simulink model "gm_Tx_OFDM"  (R2023a)
settings: Solver=FixedStepAuto  StartTime=0.0  StopTime=inf  RelTol=1e-3  EnableMultiTasking=on
model workspace (MAT data in the model file):
  M_ary = 16
  N = 64
  N_out = 256
  bit_per_symbol = 4
  fsc = 10000
  fsp = 640000
  stime = 0.0001
libraries: simulink x7, hdlmdlgenlib x4, dspsigops x4, hdlsllib x2, whdlmod x2, commdigbbndam3 x2, commrandsrc3 x1
settings Model: Creator=acer  LastModifiedBy=acer
settings SolverCC: AutoInsertRateTranBlk=on
settings OptimizationCC: BlockReduction=off  ConditionallyExecuteInputs=off  EnhancedBackFolding=on  PassReuseOutputArgsAs=Individual arguments  ZeroExternalMemoryAtStartup=off  ZeroInternalMemoryAtStartup=off  MaxStackSize=64  OptimizeBlockOrder=speed  DifferentSizesBufferReuse=on  OptimizationCustomize=off  EfficientTunableParamExpr=on
settings DebuggingCC: InheritedTsInSrcMsg=none  SingleTaskRateTransMsg=error  ParameterTunabilityLossMsg=error
settings HardwareCC: ProdBitPerPointer=32  ProdBitPerSizeT=32  ProdBitPerPtrDiffT=32  ProdLargestAtomicInteger=Long  ProdLargestAtomicFloat=Double  ProdWordSize=32  ProdHWDeviceType=ARM Compatible->ARM Cortex
settings SFSimCC: MATLABDynamicMemAlloc=off
settings RTWCC: Description=Embedded Coder  SystemTargetFile=ert.tlc  TLCOptions="-aInlineSetEventsForThisBaseRateFcn=TLC_FALSE -aSuppressMultiTaskScheduler=TLC_FALSE  -aRateBasedStepFcn=0"  TemplateMakefile=ert_default_tmf
settings CodeAppCC: ForceParamTrailComments=on  IgnoreCustomStorageClasses=off  OperatorAnnotations=on  SimulinkDataObjDesc=on  SFDataObjDesc=on  InsertBlockDesc=on

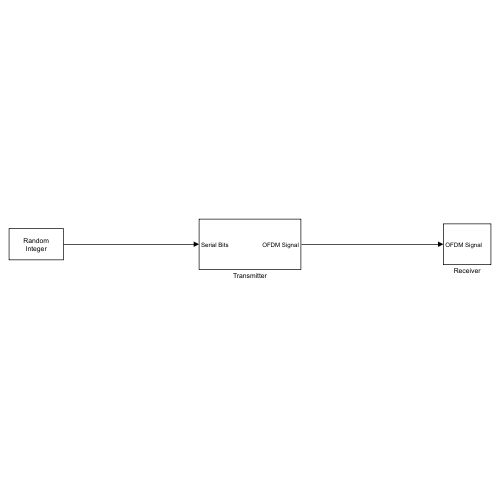
[thumbnail: Simulink's stored preview of the top-level diagram]
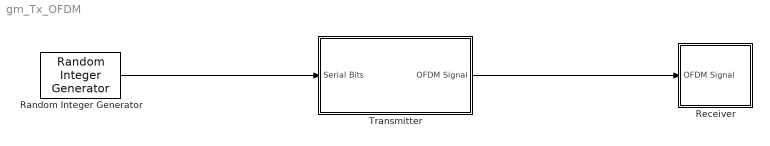
== system gm_Tx_OFDM ==
  Random Integer Generator : commrandsrc3/Random Integer Generator  SetSize=16  SeedSource=Auto  Seed=0  SampleTime=stime  SamplesPerFrame=1  OutputDataType=uint8  SimulateUsing=Interpreted execution
  Receiver : Subsystem
  Transmitter : Subsystem
  wires:
  Random Integer Generator/1 -> Transmitter/1(Serial Bits)
  Transmitter/1(OFDM Signal) -> Receiver/1(OFDM Signal)

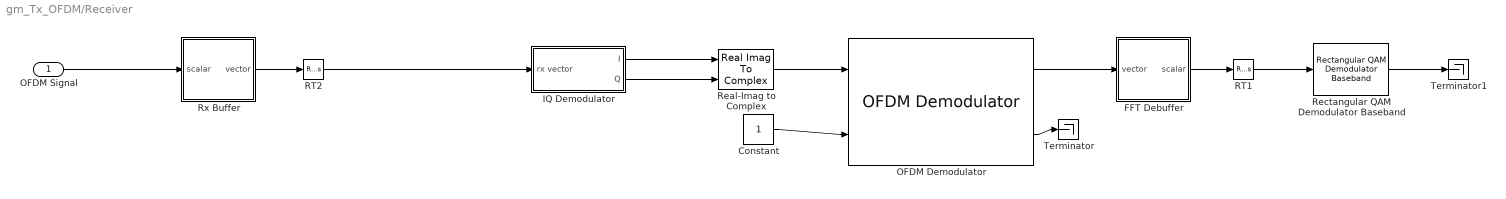
== system gm_Tx_OFDM/Receiver ==
  OFDM Signal : Inport
  Constant : Constant  OutDataTypeStr=boolean  SampleTime=-1
  FFT Debuffer : Subsystem
  IQ Demodulator : Subsystem
  OFDM Demodulator : whdlmod/OFDM Demodulator  OFDMParamsSource=Property  MaxFFTLength=64  FFTLength=N*2  CPLength=32  NumLGsC=16  NumRGsC=15  CPFraction=off  CPFractionSource=Property  CPFractionValue=0.55  removeDCSubcarriers=on  enableResetInputPort=off  Normalize=off  RoundingMethod=Floor  SimulateUsing=Code generation
  RT1 : RateTransition  OutPortSampleTime=stime/N
  RT2 : RateTransition  OutPortSampleTime=stime
  Real-Imag to Complex : RealImagToComplex
  Rectangular QAM Demodulator Baseband : commdigbbndam3/Rectangular QAM Demodulator Baseband  M=16  OutType=Integer  DecType=Hard decision  VarSource=Dialog  Variance=1  Dec=Gray  Mapping=[0:15]  PowType=Min. distance between symbols  MinDist=2  AvgPow=1  PeakPow=1  Ph=0  outDtype1=Inherit via internal rule  outDtype2=Inherit via internal rule  derotateFactorWordLen=16  derotateFactorDataTypeStr=Inherit: Same word length as input  derotateFactorLastDataTypeStr=Inherit: Same word length as input  denormFactorWordLen=16  denormFactorDataTypeStr=Inherit: Same word length as input  denormFactorLastDataTypeStr=Inherit: Same word length as input  prodOutWordLen=32  prodOutOverflowMode=Wrap  prodOutRoundingMode=Floor  prodOutOvFlMode=off  prodOutOvFlModeLastStrValue=off  sumWordLen=32
      settings: LibrarySourceBlock=|
      | commhdldigbbndam/Rectangular QAM
      | Demodulator
      | Baseband
  Rx Buffer : Subsystem
  Terminator : Terminator
  Terminator1 : Terminator
  wires:
  IQ Demodulator/2(Q) -> Real-Imag to Complex/2
  IQ Demodulator/1(I) -> Real-Imag to Complex/1
  RT2/1 -> IQ Demodulator/1(rx vector)
  Rectangular QAM Demodulator Baseband/1 -> Terminator1/1
  RT1/1 -> Rectangular QAM Demodulator Baseband/1
  FFT Debuffer/1(scalar) -> RT1/1
  OFDM Demodulator/1 -> FFT Debuffer/1(vector)
  OFDM Demodulator/2 -> Terminator/1
  Constant/1 -> OFDM Demodulator/2
  Real-Imag to Complex/1 -> OFDM Demodulator/1
  Rx Buffer/1(vector) -> RT2/1
  OFDM Signal/1 -> Rx Buffer/1(scalar)

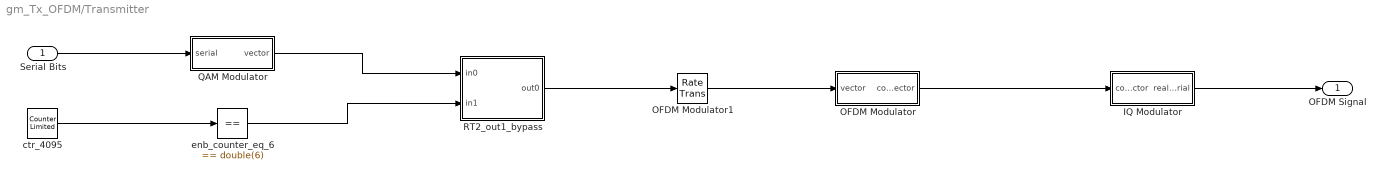
== system gm_Tx_OFDM/Transmitter ==
  Serial Bits : Inport  OutDataTypeStr=uint8  PortDimensions=1  SampleTime=0.0001
  IQ Modulator : Subsystem
  OFDM Modulator : Subsystem
  OFDM Modulator1 : RateTransition  OutPortSampleTimeOpt=Multiple of input port sample time  OutPortSampleTimeMultiple=4096
  QAM Modulator : Subsystem
  RT2_out1_bypass : Subsystem
  ctr_4095 : simulink/Sources/Counter Limited  uplimit=double(4095)  tsamp=1.5625e-06
  enb_counter_eq_6 : simulink/Logic and Bit Operations/Compare To Constant  relop===  const=double(6)  OutDataTypeStr=boolean
  OFDM Signal : Outport  SampleTime=1.5625e-06
  wires:
  Serial Bits/1 -> QAM Modulator/1(serial)
  IQ Modulator/1(real_serial) -> OFDM Signal/1
  OFDM Modulator/1(complex_vector) -> IQ Modulator/1(complex_vector)
  QAM Modulator/1(vector) -> RT2_out1_bypass/1(in0)
  OFDM Modulator1/1 -> OFDM Modulator/1(vector)
  RT2_out1_bypass/1(out0) -> OFDM Modulator1/1
  enb_counter_eq_6/1 -> RT2_out1_bypass/2(in1)
  ctr_4095/1 -> enb_counter_eq_6/1

== system gm_Tx_OFDM/Receiver/FFT Debuffer ==
  note: When changing N, change the vector init size to N manually
  vector : Inport
  Data Type Conversion : DataTypeConversion  OutMin=0  OutMax=1  OutDataTypeStr=fixdt(1,16)  SaturateOnIntegerOverflow=off  RndMeth=Floor
  Data Type Conversion1 : DataTypeConversion  OutMin=0  OutMax=1  OutDataTypeStr=fixdt(1,16)  SaturateOnIntegerOverflow=off  RndMeth=Floor
  Delay : Delay  DelayLength=1
  HDL Counter : hdlsllib/Sources/HDL Counter  CountType=Count limited  CountInit=1  CountStep=1  CountMax=N  CountFromType=Initial value  CountFrom=1  CountResetPort=off  CountLoadPort=off  CountEnbPort=off  CountDirPort=off  CountHitOutputPort=off  CountDataType=Signed  CountWordLen=16  CountFracLen=0  CountSampTime=stime
  debuffer : MATLAB Function  TreatAsAtomicUnit=on
  vector feedback : MATLAB Function  TreatAsAtomicUnit=on
  scalar : Outport
  wires:
  Data Type Conversion1/1 -> debuffer/1(vector_in)
  vector/1 -> Data Type Conversion1/1
  Delay/1 -> vector feedback/1(vector_before)
  vector feedback/1(y) -> Data Type Conversion/1
  debuffer/2(vector_current) -> Delay/1
  Data Type Conversion/1 -> debuffer/3(vector_before)
  HDL Counter/1 -> debuffer/2(counter)
  debuffer/1(buffer) -> scalar/1

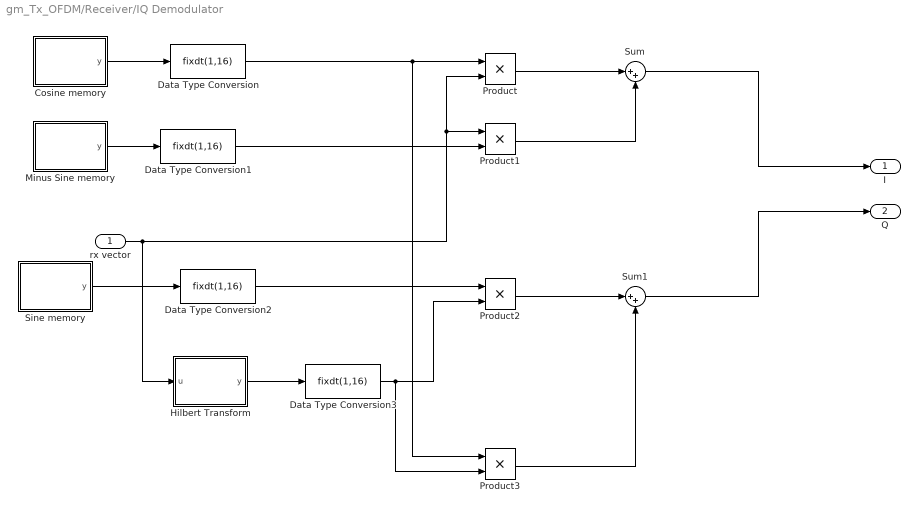
== system gm_Tx_OFDM/Receiver/IQ Demodulator ==
  rx vector : Inport
  Cosine memory : MATLAB Function  TreatAsAtomicUnit=on
  Data Type Conversion{,1..3} (4 alike) : DataTypeConversion  OutMin=0  OutMax=1  OutDataTypeStr=fixdt(1,16)  SaturateOnIntegerOverflow=off  RndMeth=Floor
  Hilbert Transform : MATLAB Function  TreatAsAtomicUnit=on
  Minus Sine memory : MATLAB Function  TreatAsAtomicUnit=on
  Product{,1..3} (4 alike) : Product
  Sine memory : MATLAB Function  TreatAsAtomicUnit=on
  Sum : Sum  Inputs=|++
  Sum1 : Sum  Inputs=|++
  I : Outport
  Q : Outport  Port=2
  wires:
  Data Type Conversion3/1 -> Product2/2, Product3/2
  Hilbert Transform/1(y) -> Data Type Conversion3/1
  Data Type Conversion2/1 -> Product2/1
  Sine memory/1(y) -> Data Type Conversion2/1
  Data Type Conversion1/1 -> Product1/2
  Minus Sine memory/1(y) -> Data Type Conversion1/1
  Data Type Conversion/1 -> Product/1, Product3/1
  Cosine memory/1(y) -> Data Type Conversion/1
  Sum/1 -> I/1
  Product3/1 -> Sum1/2
  Product2/1 -> Sum1/1
  Product/1 -> Sum/1
  Product1/1 -> Sum/2
  rx vector/1 -> Hilbert Transform/1(u), Product/2, Product1/1
  Sum1/1 -> Q/1

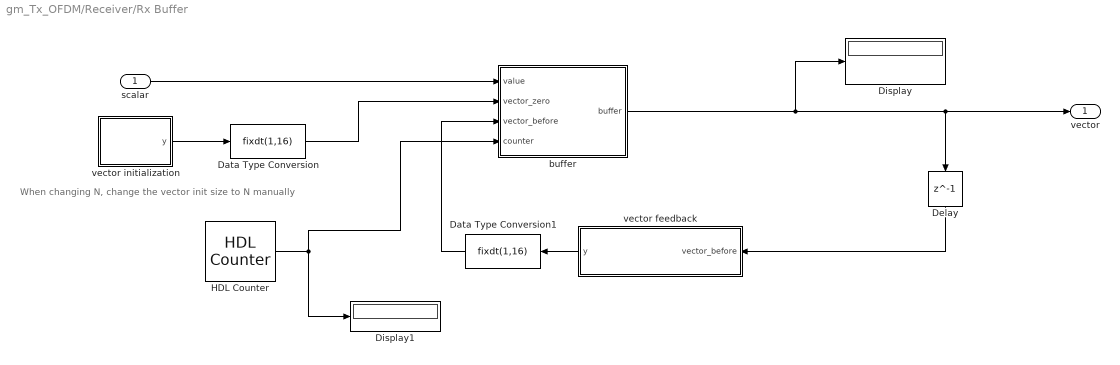
== system gm_Tx_OFDM/Receiver/Rx Buffer ==
  note: When changing N, change the vector init size to N manually
  scalar : Inport
  Data Type Conversion : DataTypeConversion  OutMin=0  OutMax=1  OutDataTypeStr=fixdt(1,16)  SaturateOnIntegerOverflow=off  RndMeth=Floor
  Data Type Conversion1 : DataTypeConversion  OutMin=0  OutMax=1  OutDataTypeStr=fixdt(1,16)  SaturateOnIntegerOverflow=off  RndMeth=Floor
  Delay : Delay  DelayLength=1
  Display : Display
  Display1 : Display
  HDL Counter : hdlsllib/Sources/HDL Counter  CountType=Count limited  CountInit=1  CountStep=1  CountMax=N  CountFromType=Initial value  CountFrom=1  CountResetPort=off  CountLoadPort=off  CountEnbPort=off  CountDirPort=off  CountHitOutputPort=off  CountDataType=Unsigned  CountWordLen=16  CountFracLen=0  CountSampTime=stime/N
  buffer : MATLAB Function  TreatAsAtomicUnit=on
  vector feedback : MATLAB Function  TreatAsAtomicUnit=on
  vector initialization : MATLAB Function  TreatAsAtomicUnit=on
  vector : Outport
  wires:
  HDL Counter/1 -> Display1/1, buffer/4(counter)
  scalar/1 -> buffer/1(value)
  Data Type Conversion1/1 -> buffer/3(vector_before)
  vector feedback/1(y) -> Data Type Conversion1/1
  Delay/1 -> vector feedback/1(vector_before)
  buffer/1(buffer) -> vector/1, Delay/1, Display/1
  Data Type Conversion/1 -> buffer/2(vector_zero)
  vector initialization/1(y) -> Data Type Conversion/1

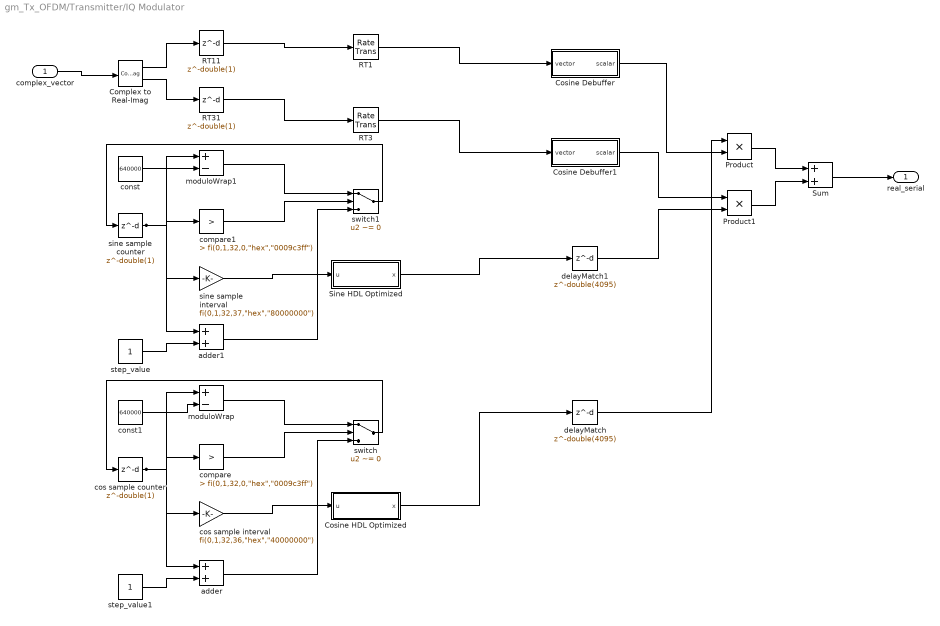
== system gm_Tx_OFDM/Transmitter/IQ Modulator ==
  complex_vector : Inport  OutDataTypeStr=fixdt(1, 16, 14)  PortDimensions=[64 1]  SampleTime=0.0064
      settings: SignalType=complex
  Complex to Real-Imag : ComplexToRealImag  SampleTime=0.0064
  Cosine Debuffer : Subsystem
  Cosine Debuffer1 : Subsystem
  Cosine HDL Optimized : Subsystem  mask(Sine and Cosine HDL optimized block){OutputFormula=cos(2*pi*u), NumDataPoints=double(64), TableDataTypeStr=fixdt(0,16,15), SimulateLUTROMDelay=off}
      mask prompts: OutputFormula "Simulink:masks:OutputFormula_MP"; NumDataPoints "HDLShared:hdlshared:CosineHDL_Npts"; TableDataTypeStr "Simulink:blkprm_prompts:TABLE_UNIFIEDDATATYPE"; SimulateLUTROMDelay "HDLShared:hdlshared:CosineHDL_SimulateLUTDelay"
      mask help: Sine and Cosine HDL optimized block using quarter wave symmetry, and HDL friendly settings.
      mask Help: helpview([docroot '/hdlcoder/helptargets.map'],'SineAndCosineHDL_Optimized');
      mask TypeOptions OutputFormula: sin(2*pi*u) | cos(2*pi*u) | exp(j*2*pi*u) | sin(2*pi*u) and cos(2*pi*u)
      mask Display:
      | port_label('input',1,'u')
      | port_label('output',1,'cos(2*pi*u)')
      | xpos = 0.35;
      | yoffset = 0.5;
      | if ( SimulateLUTROMDelay )
      |   text(xpos,yoffset,'HDL (Z^{-1})','texmode','on')
      | else
      |    text(xpos,yoffset,'HDL')
      | end
  Product : Product  Inputs=**  OutDataTypeStr=fixdt(1, 33, 29)  SampleTime=1.5625e-06
  Product1 : Product  Inputs=**  OutDataTypeStr=int16  SampleTime=1.5625e-06
  RT1 : RateTransition  Integrity=off  Deterministic=off  InitialCondition=double(0)  OutPortSampleTimeOpt=Multiple of input port sample time  OutPortSampleTimeMultiple=1/4096
  RT11 : Delay  DelayLength=double(1)  InitialCondition=0  SampleTime=0.0064
  RT3 : RateTransition  Integrity=off  Deterministic=off  InitialCondition=double(0)  OutPortSampleTimeOpt=Multiple of input port sample time  OutPortSampleTimeMultiple=1/4096
  RT31 : Delay  DelayLength=double(1)  InitialCondition=0  SampleTime=0.0064
  Sine HDL Optimized : Subsystem  mask(Sine and Cosine HDL optimized block){OutputFormula=sin(2*pi*u), NumDataPoints=double(64), TableDataTypeStr=fixdt(0,16,15), SimulateLUTROMDelay=off}
      mask prompts: OutputFormula "Simulink:masks:OutputFormula_MP"; NumDataPoints "HDLShared:hdlshared:CosineHDL_Npts"; TableDataTypeStr "Simulink:blkprm_prompts:TABLE_UNIFIEDDATATYPE"; SimulateLUTROMDelay "HDLShared:hdlshared:CosineHDL_SimulateLUTDelay"
      mask help: Sine and Cosine HDL optimized block using quarter wave symmetry, and HDL friendly settings.
      mask Help: helpview([docroot '/hdlcoder/helptargets.map'],'SineAndCosineHDL_Optimized');
      mask TypeOptions OutputFormula: sin(2*pi*u) | cos(2*pi*u) | exp(j*2*pi*u) | sin(2*pi*u) and cos(2*pi*u)
      mask Display:
      | port_label('input',1,'u')
      | port_label('output',1,'sin(2*pi*u)')
      | xpos = 0.35;
      | yoffset = 0.5;
      | if ( SimulateLUTROMDelay )
      |   text(xpos,yoffset,'HDL (Z^{-1})','texmode','on')
      | else
      |    text(xpos,yoffset,'HDL')
      | end
  Sum : Sum  AccumDataTypeStr=fixdt(1, 64, 29)  OutDataTypeStr=fixdt(1, 64, 29)  SampleTime=1.5625e-06
  adder : Sum  AccumDataTypeStr=int32  OutDataTypeStr=int32  SampleTime=1.5625e-06
  adder1 : Sum  AccumDataTypeStr=int32  OutDataTypeStr=int32  SampleTime=1.5625e-06
  compare : simulink/Logic and Bit Operations/Compare To Constant  relop=>  const="fi(0,1,32,0,\"hex\",\"0009c3ff\")"  OutDataTypeStr=boolean
  compare1 : simulink/Logic and Bit Operations/Compare To Constant  relop=>  const="fi(0,1,32,0,\"hex\",\"0009c3ff\")"  OutDataTypeStr=boolean
  const : Constant  Value=640000  VectorParams1D=off  OutDataTypeStr=int32  SampleTime=1.5625e-06
  const1 : Constant  Value=640000  VectorParams1D=off  OutDataTypeStr=int32  SampleTime=1.5625e-06
  cos sample counter : Delay  DelayLength=double(1)  InitialCondition=0  SampleTime=1.5625e-06
  cos sample interval : Gain  Gain="fi(0,1,32,36,\"hex\",\"40000000\")"  ParamDataTypeStr=fixdt(1, 32, 36)  OutDataTypeStr=fixdt(1, 64, 36)  SampleTime=1.5625e-06
  delayMatch : Delay  DelayLength=double(4095)  InitialCondition=0  SampleTime=1.5625e-06
  delayMatch1 : Delay  DelayLength=double(4095)  InitialCondition=0  SampleTime=1.5625e-06
  moduloWrap : Sum  Inputs=+-  AccumDataTypeStr=int32  OutDataTypeStr=int32  SampleTime=1.5625e-06
  moduloWrap1 : Sum  Inputs=+-  AccumDataTypeStr=int32  OutDataTypeStr=int32  SampleTime=1.5625e-06
  sine sample counter : Delay  DelayLength=double(1)  InitialCondition=0  SampleTime=1.5625e-06
  sine sample interval : Gain  Gain="fi(0,1,32,37,\"hex\",\"80000000\")"  ParamDataTypeStr=fixdt(1, 32, 37)  OutDataTypeStr=fixdt(1, 64, 37)  SampleTime=1.5625e-06
  step_value : Constant  VectorParams1D=off  OutDataTypeStr=int32  SampleTime=1.5625e-06
  step_value1 : Constant  VectorParams1D=off  OutDataTypeStr=int32  SampleTime=1.5625e-06
  switch : Switch  Criteria=u2 ~= 0  Threshold=double(0)  OutDataTypeStr=int32  SampleTime=1.5625e-06  SaturateOnIntegerOverflow=off  InputSameDT=off
  switch1 : Switch  Criteria=u2 ~= 0  Threshold=double(0)  OutDataTypeStr=int32  SampleTime=1.5625e-06  SaturateOnIntegerOverflow=off  InputSameDT=off
  real_serial : Outport  SampleTime=1.5625e-06
  wires:
  Cosine Debuffer/1(scalar) -> Product/2
  Cosine Debuffer1/1(scalar) -> Product1/1
  Sum/1 -> real_serial/1
  cos sample counter/1 -> cos sample interval/1, compare/1, moduloWrap/1, adder/1
  sine sample counter/1 -> sine sample interval/1, compare1/1, moduloWrap1/1, adder1/1
  RT1/1 -> Cosine Debuffer/1(vector)
  RT3/1 -> Cosine Debuffer1/1(vector)
  RT11/1 -> RT1/1
  RT31/1 -> RT3/1
  sine sample interval/1 -> Sine HDL Optimized/1(u)
  delayMatch1/1 -> Product1/2
  Product1/1 -> Sum/2
  Product/1 -> Sum/1
  cos sample interval/1 -> Cosine HDL Optimized/1(u)
  delayMatch/1 -> Product/1
  const/1 -> moduloWrap1/2
  step_value/1 -> adder1/2
  const1/1 -> moduloWrap/2
  step_value1/1 -> adder/2
  Complex to Real-Imag/1 -> RT11/1
  Complex to Real-Imag/2 -> RT31/1
  complex_vector/1 -> Complex to Real-Imag/1
  Cosine HDL Optimized/1(x) -> delayMatch/1
  Sine HDL Optimized/1(x) -> delayMatch1/1
  switch1/1 -> sine sample counter/1
  adder1/1 -> switch1/3
  compare1/1 -> switch1/2
  moduloWrap1/1 -> switch1/1
  switch/1 -> cos sample counter/1
  adder/1 -> switch/3
  compare/1 -> switch/2
  moduloWrap/1 -> switch/1

== system gm_Tx_OFDM/Transmitter/OFDM Modulator ==
  vector : Inport  OutDataTypeStr=fixdt(1, 16, 14)  PortDimensions=[64]  SampleTime=0.0064
      settings: SignalType=complex
  Constant : Constant  OutDataTypeStr=boolean  SampleTime=0.0064
  OFDM Modulator : Subsystem
  complex_vector : Outport  SampleTime=0.0064
  wires:
  Constant/1 -> OFDM Modulator/2(valid)
  OFDM Modulator/1(data1) -> complex_vector/1
  vector/1 -> OFDM Modulator/1(data)

== system gm_Tx_OFDM/Transmitter/QAM Modulator ==
  note: When changing N, change the vector init size to N manually
  serial : Inport  OutDataTypeStr=uint8  PortDimensions=1  SampleTime=0.0001
  QAM Buffer : Subsystem
  Rectangular QAM Modulator Baseband : commdigbbndam3/Rectangular QAM Modulator Baseband  M=M_ary  InType=Integer  Enc=Gray  Mapping=[0:15]  PowType=Min. distance between symbols  MinDist=2  AvgPow=1  PeakPow=1  Ph=0  outDtype=Fixed-point  outWordLen=16  outUDDataType=sfix(16)  outFracLenMode=Best precision  outFracLen=15  outDataTypeStr=fixdt(1,16)  outLastDataTypeStr=fixdt(1,16)
      settings: LibrarySourceBlock=|
      | commhdldigbbndam/Rectangular QAM
      | Modulator
      | Baseband
  vector : Outport  SampleTime=1.5625e-06
  wires:
  Rectangular QAM Modulator Baseband/1 -> QAM Buffer/1(scalar)
  QAM Buffer/1(vector) -> vector/1
  serial/1 -> Rectangular QAM Modulator Baseband/1

== system gm_Tx_OFDM/Transmitter/RT2_out1_bypass ==
  in0 : Inport  OutDataTypeStr=fixdt(1,16,14,'DataTypeOverride', 'Off')  PortDimensions=[64]  SampleTime=1.5625e-06
      settings: SignalType=complex
  in1 : Inport  Port=2  OutDataTypeStr=boolean  SampleTime=1.5625e-06
  RT2_out1_enb : Switch  Criteria=u2 ~= 0  Threshold=double(0)  OutDataTypeStr=fixdt(1, 16, 14)  SampleTime=1.5625e-06  SaturateOnIntegerOverflow=off  InputSameDT=off
  RT2_out1_state : Delay  DelayLength=double(1)  InitialCondition=0  SampleTime=1.5625e-06
  out0 : Outport  OutDataTypeStr=fixdt(1, 16, 14)  PortDimensions=[64]  SampleTime=1.5625e-06
      settings: SignalType=complex
  wires:
  RT2_out1_enb/1 -> out0/1, RT2_out1_state/1
  in0/1 -> RT2_out1_enb/1
  in1/1 -> RT2_out1_enb/2
  RT2_out1_state/1 -> RT2_out1_enb/3

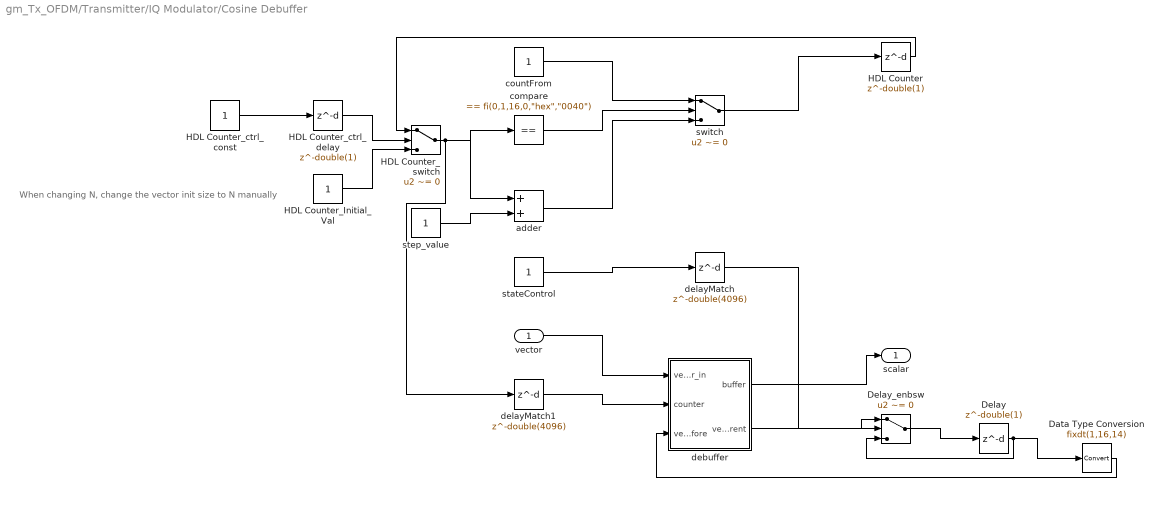
== system gm_Tx_OFDM/Transmitter/IQ Modulator/Cosine Debuffer ==
  note: When changing N, change the vector init size to N manually
  vector : Inport  OutDataTypeStr=fixdt(1, 16, 14)  PortDimensions=[64 1]  SampleTime=1.5625e-06
  Data Type Conversion : DataTypeConversion  OutDataTypeStr=fixdt(1,16,14)
  Delay : Delay  DelayLength=double(1)  InitialCondition=0  SampleTime=1.5625e-06
  Delay_enbsw : Switch  Criteria=u2 ~= 0  Threshold=double(0)  OutDataTypeStr=fixdt(1, 16, 14)  SampleTime=1.5625e-06  SaturateOnIntegerOverflow=off  InputSameDT=off
  HDL Counter : Delay  DelayLength=double(1)  InitialCondition=0  SampleTime=1.5625e-06
  HDL Counter_Initial_Val : Constant  OutDataTypeStr=int16  SampleTime=1.5625e-06
  HDL Counter_ctrl_const : Constant  OutDataTypeStr=boolean  SampleTime=1.5625e-06
  HDL Counter_ctrl_delay : Delay  DelayLength=double(1)  InitialCondition=0  SampleTime=1.5625e-06
  HDL Counter_switch : Switch  Criteria=u2 ~= 0  Threshold=double(0)  OutDataTypeStr=int16  SampleTime=1.5625e-06  SaturateOnIntegerOverflow=off  InputSameDT=off
  adder : Sum  AccumDataTypeStr=int16  OutDataTypeStr=int16  SampleTime=1.5625e-06
  compare : simulink/Logic and Bit Operations/Compare To Constant  relop===  const="fi(0,1,16,0,\"hex\",\"0040\")"  OutDataTypeStr=boolean
  countFrom : Constant  VectorParams1D=off  OutDataTypeStr=int16  SampleTime=1.5625e-06
  debuffer : Subsystem
  delayMatch : Delay  DelayLength=double(4096)  InitialCondition=0  SampleTime=1.5625e-06
  delayMatch1 : Delay  DelayLength=double(4096)  InitialCondition=0  SampleTime=1.5625e-06
  stateControl : Constant  OutDataTypeStr=boolean  SampleTime=1.5625e-06
  step_value : Constant  VectorParams1D=off  OutDataTypeStr=int16  SampleTime=1.5625e-06
  switch : Switch  Criteria=u2 ~= 0  Threshold=double(0)  OutDataTypeStr=int16  SampleTime=1.5625e-06  SaturateOnIntegerOverflow=off  InputSameDT=off
  scalar : Outport  SampleTime=1.5625e-06
  wires:
  delayMatch1/1 -> debuffer/2(counter)
  step_value/1 -> adder/2
  countFrom/1 -> switch/1
  HDL Counter_Initial_Val/1 -> HDL Counter_switch/3
  HDL Counter_ctrl_const/1 -> HDL Counter_ctrl_delay/1
  HDL Counter_ctrl_delay/1 -> HDL Counter_switch/2
  delayMatch/1 -> Delay_enbsw/2
  vector/1 -> debuffer/1(vector_in)
  stateControl/1 -> delayMatch/1
  HDL Counter_switch/1 -> delayMatch1/1, adder/1, compare/1
  HDL Counter/1 -> HDL Counter_switch/1
  switch/1 -> HDL Counter/1
  adder/1 -> switch/3
  compare/1 -> switch/2
  Delay/1 -> Data Type Conversion/1, Delay_enbsw/3
  Data Type Conversion/1 -> debuffer/3(vector_before)
  debuffer/2(vector_current) -> Delay_enbsw/1
  debuffer/1(buffer) -> scalar/1
  Delay_enbsw/1 -> Delay/1

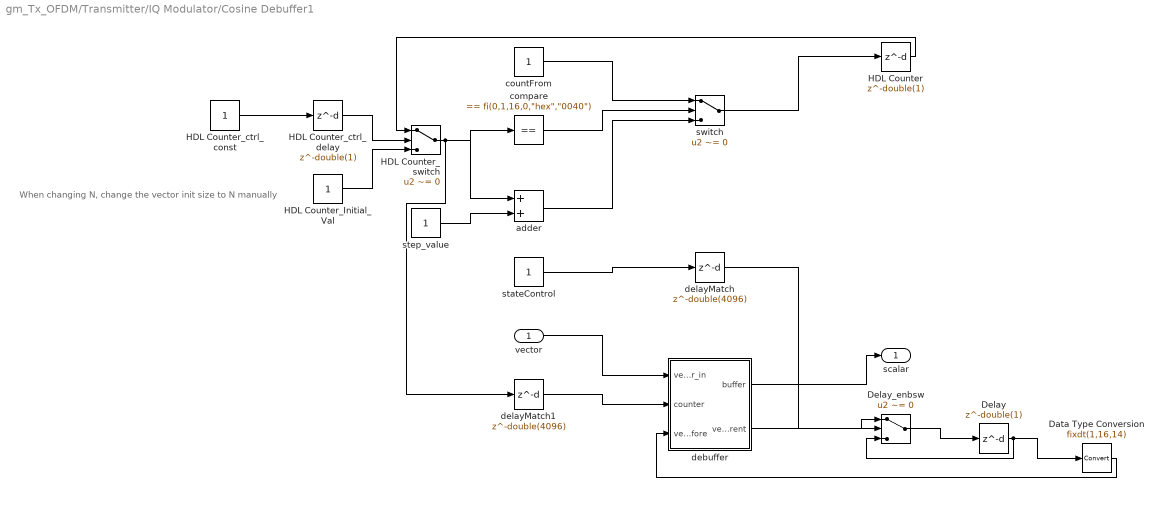
== system gm_Tx_OFDM/Transmitter/IQ Modulator/Cosine Debuffer1 ==
  note: When changing N, change the vector init size to N manually
  vector : Inport  OutDataTypeStr=fixdt(1, 16, 14)  PortDimensions=[64 1]  SampleTime=1.5625e-06
  Data Type Conversion : DataTypeConversion  OutDataTypeStr=fixdt(1,16,14)
  Delay : Delay  DelayLength=double(1)  InitialCondition=0  SampleTime=1.5625e-06
  Delay_enbsw : Switch  Criteria=u2 ~= 0  Threshold=double(0)  OutDataTypeStr=fixdt(1, 16, 14)  SampleTime=1.5625e-06  SaturateOnIntegerOverflow=off  InputSameDT=off
  HDL Counter : Delay  DelayLength=double(1)  InitialCondition=0  SampleTime=1.5625e-06
  HDL Counter_Initial_Val : Constant  OutDataTypeStr=int16  SampleTime=1.5625e-06
  HDL Counter_ctrl_const : Constant  OutDataTypeStr=boolean  SampleTime=1.5625e-06
  HDL Counter_ctrl_delay : Delay  DelayLength=double(1)  InitialCondition=0  SampleTime=1.5625e-06
  HDL Counter_switch : Switch  Criteria=u2 ~= 0  Threshold=double(0)  OutDataTypeStr=int16  SampleTime=1.5625e-06  SaturateOnIntegerOverflow=off  InputSameDT=off
  adder : Sum  AccumDataTypeStr=int16  OutDataTypeStr=int16  SampleTime=1.5625e-06
  compare : simulink/Logic and Bit Operations/Compare To Constant  relop===  const="fi(0,1,16,0,\"hex\",\"0040\")"  OutDataTypeStr=boolean
  countFrom : Constant  VectorParams1D=off  OutDataTypeStr=int16  SampleTime=1.5625e-06
  debuffer : Subsystem
  delayMatch : Delay  DelayLength=double(4096)  InitialCondition=0  SampleTime=1.5625e-06
  delayMatch1 : Delay  DelayLength=double(4096)  InitialCondition=0  SampleTime=1.5625e-06
  stateControl : Constant  OutDataTypeStr=boolean  SampleTime=1.5625e-06
  step_value : Constant  VectorParams1D=off  OutDataTypeStr=int16  SampleTime=1.5625e-06
  switch : Switch  Criteria=u2 ~= 0  Threshold=double(0)  OutDataTypeStr=int16  SampleTime=1.5625e-06  SaturateOnIntegerOverflow=off  InputSameDT=off
  scalar : Outport  SampleTime=1.5625e-06
  wires:
  delayMatch1/1 -> debuffer/2(counter)
  step_value/1 -> adder/2
  countFrom/1 -> switch/1
  HDL Counter_Initial_Val/1 -> HDL Counter_switch/3
  HDL Counter_ctrl_const/1 -> HDL Counter_ctrl_delay/1
  HDL Counter_ctrl_delay/1 -> HDL Counter_switch/2
  delayMatch/1 -> Delay_enbsw/2
  vector/1 -> debuffer/1(vector_in)
  stateControl/1 -> delayMatch/1
  HDL Counter_switch/1 -> delayMatch1/1, adder/1, compare/1
  HDL Counter/1 -> HDL Counter_switch/1
  switch/1 -> HDL Counter/1
  adder/1 -> switch/3
  compare/1 -> switch/2
  Delay/1 -> Data Type Conversion/1, Delay_enbsw/3
  Data Type Conversion/1 -> debuffer/3(vector_before)
  debuffer/2(vector_current) -> Delay_enbsw/1
  debuffer/1(buffer) -> scalar/1
  Delay_enbsw/1 -> Delay/1

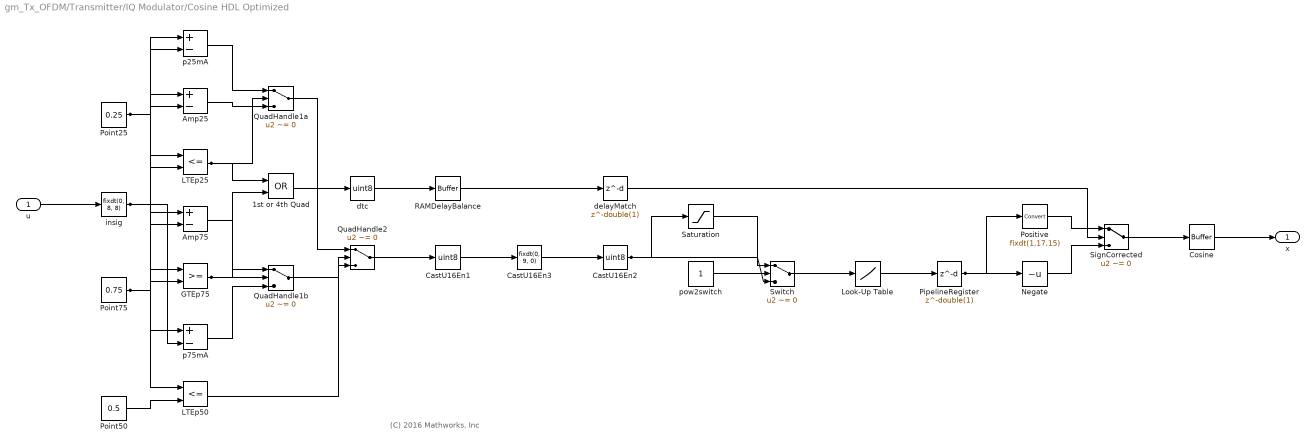
== system gm_Tx_OFDM/Transmitter/IQ Modulator/Cosine HDL Optimized ==
  note: (C) 2016 Mathworks, Inc
  u : Inport  OutDataTypeStr=fixdt(1,64,36,'DataTypeOverride', 'Off')  SampleTime=1.5625e-06
  1st or 4th Quad : Logic  Operator=OR  AllPortsSameDT=off  OutDataTypeStr=boolean  SampleTime=1.5625e-06
  Amp25 : Sum  Inputs=+-  AccumDataTypeStr=fixdt(1, 32, 17)  OutDataTypeStr=fixdt(0, 32, 17)  SampleTime=1.5625e-06
  Amp75 : Sum  Inputs=+-  AccumDataTypeStr=fixdt(1, 32, 17)  OutDataTypeStr=fixdt(0, 32, 17)  SampleTime=1.5625e-06
  CastU16En1 : DataTypeConversion  OutDataTypeStr=uint8  ConvertRealWorld=Stored Integer (SI)  SampleTime=1.5625e-06  SaturateOnIntegerOverflow=off  RndMeth=Floor
  CastU16En2 : DataTypeConversion  OutDataTypeStr=uint8  ConvertRealWorld=Stored Integer (SI)  SampleTime=1.5625e-06  RndMeth=Floor
  CastU16En3 : DataTypeConversion  OutDataTypeStr=fixdt(0, 9, 0)  SampleTime=1.5625e-06  SaturateOnIntegerOverflow=off  RndMeth=Floor
  Cosine : hdlmdlgenlib/Buffer
  GTEp75 : RelationalOperator  OutDataTypeStr=boolean  SampleTime=1.5625e-06  InputSameDT=off
  LTEp25 : RelationalOperator  Operator=<=  OutDataTypeStr=boolean  SampleTime=1.5625e-06  InputSameDT=off
  LTEp50 : RelationalOperator  Operator=<=  OutDataTypeStr=boolean  SampleTime=1.5625e-06  InputSameDT=off
  Look-Up Table : Lookup_n-D  NumberOfTableDimensions=1  BreakpointsForDimension1="fi(\"numerictype\",numerictype(0,8,0),\"fimath\",fimath(\"RoundingMethod\", \"Floor\",\"OverflowAction\", \"Wrap\",\"ProductMode\",\"FullPrecision\",\"SumMode\",\"FullPrecision\"),\"Value\",\"[0 1 2 3 4 5 6 7 8 9 10 11 12 13 14 15 16 17 18 19 20 21 22 23 24 25 26 27 28 29 30 31 32 33 34 35 36 37 38 39 40 41 42 43 44 45 46 47 48 49 50 51 52 53 54 55 56 57 58 59 60 61 62 63]\")"  Table="reshape(fi(\"numerictype\",numerictype(1,17,15),\"fimath\",fimath(\"RoundingMethod\", \"Floor\",\"OverflowAction\", \"Wrap\",\"ProductMode\",\"FullPrecision\",\"SumMode\",\"FullPrecision\"),\"Value\",\"[0;0.0245361328125;0.049072265625;0.073577880859375;0.0980224609375;0.122406005859375;0.146728515625;0.17095947265625;0.195098876953125;0.2191162109375;0.24298095703125;0.2667236328125;0.290283203125;0.313690185546875;0.336883544921875;0.359893798828125;0.3826904296875;0.405242919921875;0.42755126953125;0.449615478515625;0.471405029296875;0.492889404296875;0.51409912109375;0.535003662109375;0.555572509765625;0.5758056640625;0.595703125;0.615234375;0.6343994140625;0.653167724609375;0.67156982421875;0.689544677734375;0.70709228515625;0.7242431640625;0.740936279296875;0.7572021484375;0.77301025390625;0.788360595703125;0.80322265625;0.817596435546875;0.83148193359375;0.8448486328125;0.85772705078125;0.870086669921875;0.881927490234375;0.893218994140625;0.90399169921875;0.914215087890625;0.92388916015625;0.9329833984375;0.941558837890625;0.94952392578125;0.956939697265625;0.963775634765625;0.97003173828125;0.9757080078125;0.98077392578125;0.98529052734375;0.989166259765625;0.99249267578125;0.99517822265625;0.997283935546875;0.998809814453125;0.99969482421875]\"), [1  64])"  InterpMethod=Flat  ExtrapMethod=Clip  DiagnosticForOutOfRangeInput=Error  SampleTime=1.5625e-06  OutDataTypeStr=fixdt(1, 17, 15)
  Negate : UnaryMinus  SampleTime=1.5625e-06
  PipelineRegister : Delay  DelayLength=double(1)  InitialCondition=0  SampleTime=1.5625e-06
  Point25 : Constant  Value=0.25  OutDataTypeStr=fixdt(0, 17, 17)  SampleTime=1.5625e-06
  Point50 : Constant  Value=0.5  OutDataTypeStr=fixdt(0, 17, 17)  SampleTime=1.5625e-06
  Point75 : Constant  Value=0.75  OutDataTypeStr=fixdt(0, 17, 17)  SampleTime=1.5625e-06
  Positive : DataTypeConversion  OutDataTypeStr=fixdt(1,17,15)
  QuadHandle1a : Switch  Criteria=u2 ~= 0  Threshold=double(0)  OutDataTypeStr=fixdt(0, 32, 17)  SampleTime=1.5625e-06  SaturateOnIntegerOverflow=off  InputSameDT=off
  QuadHandle1b : Switch  Criteria=u2 ~= 0  Threshold=double(0)  OutDataTypeStr=fixdt(0, 32, 17)  SampleTime=1.5625e-06  SaturateOnIntegerOverflow=off  InputSameDT=off
  QuadHandle2 : Switch  Criteria=u2 ~= 0  Threshold=double(0)  OutDataTypeStr=fixdt(0, 8, 8)  SampleTime=1.5625e-06  InputSameDT=off
  RAMDelayBalance : hdlmdlgenlib/Buffer
  Saturation : Saturate  UpperLimit="fi(0,0,8,0,\"hex\",\"3f\")"  LowerLimit="fi(0,0,8,0,\"hex\",\"00\")"  SampleTime=1.5625e-06  OutDataTypeStr=uint8
  SignCorrected : Switch  Criteria=u2 ~= 0  Threshold=double(0)  OutDataTypeStr=fixdt(1, 17, 15)  SampleTime=1.5625e-06  SaturateOnIntegerOverflow=off  InputSameDT=off
  Switch : Switch  Criteria=u2 ~= 0  Threshold=double(0)  OutDataTypeStr=uint8  SampleTime=1.5625e-06  SaturateOnIntegerOverflow=off  InputSameDT=off
  delayMatch : Delay  DelayLength=double(1)  InitialCondition=0  SampleTime=1.5625e-06
  dtc : DataTypeConversion  OutDataTypeStr=uint8  ConvertRealWorld=Stored Integer (SI)  SampleTime=1.5625e-06  SaturateOnIntegerOverflow=off  RndMeth=Floor
  insig : DataTypeConversion  OutDataTypeStr=fixdt(0, 8, 8)  SampleTime=1.5625e-06  SaturateOnIntegerOverflow=off  RndMeth=Floor
  p25mA : Sum  Inputs=+-  AccumDataTypeStr=fixdt(1, 32, 17)  OutDataTypeStr=fixdt(0, 32, 17)  SampleTime=1.5625e-06
  p75mA : Sum  Inputs=+-  AccumDataTypeStr=fixdt(1, 32, 17)  OutDataTypeStr=fixdt(0, 32, 17)  SampleTime=1.5625e-06
  pow2switch : Constant  OutDataTypeStr=boolean  SampleTime=1.5625e-06
  x : Outport  SampleTime=1.5625e-06
  wires:
  Cosine/1 -> x/1
  dtc/1 -> RAMDelayBalance/1
  Amp25/1 -> QuadHandle1a/3
  Amp75/1 -> QuadHandle1b/1
  CastU16En1/1 -> CastU16En3/1
  CastU16En2/1 -> Switch/3, Saturation/1
  CastU16En3/1 -> CastU16En2/1
  GTEp75/1 -> QuadHandle1b/2, 1st or 4th Quad/2
  LTEp25/1 -> QuadHandle1a/2, 1st or 4th Quad/1
  LTEp50/1 -> QuadHandle2/2
  PipelineRegister/1 -> Positive/1, Negate/1
  Negate/1 -> SignCorrected/3
  Point25/1 -> p25mA/1, LTEp25/2, Amp25/2
  Point50/1 -> LTEp50/2
  Point75/1 -> p75mA/1, GTEp75/2, Amp75/2
  Positive/1 -> SignCorrected/1
  QuadHandle1a/1 -> QuadHandle2/1
  QuadHandle1b/1 -> QuadHandle2/3
  QuadHandle2/1 -> CastU16En1/1
  delayMatch/1 -> SignCorrected/2
  Saturation/1 -> Switch/1
  SignCorrected/1 -> Cosine/1
  Switch/1 -> Look-Up Table/1
  insig/1 -> p75mA/2, p25mA/2, LTEp50/1, LTEp25/1, GTEp75/1, Amp75/1, Amp25/1
  p25mA/1 -> QuadHandle1a/1
  p75mA/1 -> QuadHandle1b/3
  pow2switch/1 -> Switch/2
  1st or 4th Quad/1 -> dtc/1
  u/1 -> insig/1
  RAMDelayBalance/1 -> delayMatch/1
  Look-Up Table/1 -> PipelineRegister/1

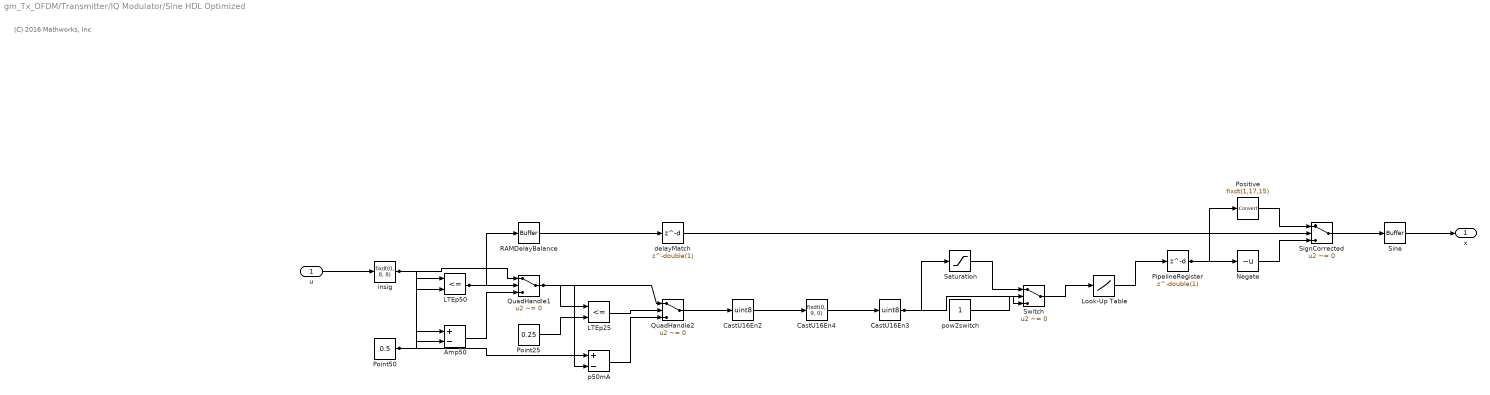
== system gm_Tx_OFDM/Transmitter/IQ Modulator/Sine HDL Optimized ==
  note: (C) 2016 Mathworks, Inc
  u : Inport  OutDataTypeStr=fixdt(1,64,37,'DataTypeOverride', 'Off')  SampleTime=1.5625e-06
  Amp50 : Sum  Inputs=+-  AccumDataTypeStr=fixdt(1, 32, 17)  OutDataTypeStr=fixdt(0, 32, 17)  SampleTime=1.5625e-06
  CastU16En2 : DataTypeConversion  OutDataTypeStr=uint8  ConvertRealWorld=Stored Integer (SI)  SampleTime=1.5625e-06  SaturateOnIntegerOverflow=off  RndMeth=Floor
  CastU16En3 : DataTypeConversion  OutDataTypeStr=uint8  ConvertRealWorld=Stored Integer (SI)  SampleTime=1.5625e-06  RndMeth=Floor
  CastU16En4 : DataTypeConversion  OutDataTypeStr=fixdt(0, 9, 0)  SampleTime=1.5625e-06  SaturateOnIntegerOverflow=off  RndMeth=Floor
  LTEp25 : RelationalOperator  Operator=<=  OutDataTypeStr=boolean  SampleTime=1.5625e-06  InputSameDT=off
  LTEp50 : RelationalOperator  Operator=<=  OutDataTypeStr=boolean  SampleTime=1.5625e-06  InputSameDT=off
  Look-Up Table : Lookup_n-D  NumberOfTableDimensions=1  BreakpointsForDimension1="fi(\"numerictype\",numerictype(0,8,0),\"fimath\",fimath(\"RoundingMethod\", \"Floor\",\"OverflowAction\", \"Wrap\",\"ProductMode\",\"FullPrecision\",\"SumMode\",\"FullPrecision\"),\"Value\",\"[0 1 2 3 4 5 6 7 8 9 10 11 12 13 14 15 16 17 18 19 20 21 22 23 24 25 26 27 28 29 30 31 32 33 34 35 36 37 38 39 40 41 42 43 44 45 46 47 48 49 50 51 52 53 54 55 56 57 58 59 60 61 62 63]\")"  Table="reshape(fi(\"numerictype\",numerictype(1,17,15),\"fimath\",fimath(\"RoundingMethod\", \"Floor\",\"OverflowAction\", \"Wrap\",\"ProductMode\",\"FullPrecision\",\"SumMode\",\"FullPrecision\"),\"Value\",\"[0;0.0245361328125;0.049072265625;0.073577880859375;0.0980224609375;0.122406005859375;0.146728515625;0.17095947265625;0.195098876953125;0.2191162109375;0.24298095703125;0.2667236328125;0.290283203125;0.313690185546875;0.336883544921875;0.359893798828125;0.3826904296875;0.405242919921875;0.42755126953125;0.449615478515625;0.471405029296875;0.492889404296875;0.51409912109375;0.535003662109375;0.555572509765625;0.5758056640625;0.595703125;0.615234375;0.6343994140625;0.653167724609375;0.67156982421875;0.689544677734375;0.70709228515625;0.7242431640625;0.740936279296875;0.7572021484375;0.77301025390625;0.788360595703125;0.80322265625;0.817596435546875;0.83148193359375;0.8448486328125;0.85772705078125;0.870086669921875;0.881927490234375;0.893218994140625;0.90399169921875;0.914215087890625;0.92388916015625;0.9329833984375;0.941558837890625;0.94952392578125;0.956939697265625;0.963775634765625;0.97003173828125;0.9757080078125;0.98077392578125;0.98529052734375;0.989166259765625;0.99249267578125;0.99517822265625;0.997283935546875;0.998809814453125;0.99969482421875]\"), [1  64])"  InterpMethod=Flat  ExtrapMethod=Clip  DiagnosticForOutOfRangeInput=Error  SampleTime=1.5625e-06  OutDataTypeStr=fixdt(1, 17, 15)
  Negate : UnaryMinus  SampleTime=1.5625e-06
  PipelineRegister : Delay  DelayLength=double(1)  InitialCondition=0  SampleTime=1.5625e-06
  Point25 : Constant  Value=0.25  OutDataTypeStr=fixdt(0, 17, 17)  SampleTime=1.5625e-06
  Point50 : Constant  Value=0.5  OutDataTypeStr=fixdt(0, 17, 17)  SampleTime=1.5625e-06
  Positive : DataTypeConversion  OutDataTypeStr=fixdt(1,17,15)
  QuadHandle1 : Switch  Criteria=u2 ~= 0  Threshold=double(0)  OutDataTypeStr=fixdt(0, 32, 17)  SampleTime=1.5625e-06  SaturateOnIntegerOverflow=off  InputSameDT=off
  QuadHandle2 : Switch  Criteria=u2 ~= 0  Threshold=double(0)  OutDataTypeStr=fixdt(0, 8, 8)  SampleTime=1.5625e-06  SaturateOnIntegerOverflow=off  InputSameDT=off
  RAMDelayBalance : hdlmdlgenlib/Buffer
  Saturation : Saturate  UpperLimit="fi(0,0,8,0,\"hex\",\"3f\")"  LowerLimit="fi(0,0,8,0,\"hex\",\"00\")"  SampleTime=1.5625e-06  OutDataTypeStr=uint8
  SignCorrected : Switch  Criteria=u2 ~= 0  Threshold=double(0)  OutDataTypeStr=fixdt(1, 17, 15)  SampleTime=1.5625e-06  SaturateOnIntegerOverflow=off  InputSameDT=off
  Sine : hdlmdlgenlib/Buffer
  Switch : Switch  Criteria=u2 ~= 0  Threshold=double(0)  OutDataTypeStr=uint8  SampleTime=1.5625e-06  SaturateOnIntegerOverflow=off  InputSameDT=off
  delayMatch : Delay  DelayLength=double(1)  InitialCondition=0  SampleTime=1.5625e-06
  insig : DataTypeConversion  OutDataTypeStr=fixdt(0, 8, 8)  SampleTime=1.5625e-06  SaturateOnIntegerOverflow=off  RndMeth=Floor
  p50mA : Sum  Inputs=+-  AccumDataTypeStr=fixdt(0, 32, 17)  OutDataTypeStr=fixdt(0, 32, 17)  SampleTime=1.5625e-06
  pow2switch : Constant  OutDataTypeStr=boolean  SampleTime=1.5625e-06
  x : Outport  SampleTime=1.5625e-06
  wires:
  Sine/1 -> x/1
  Amp50/1 -> QuadHandle1/3
  CastU16En2/1 -> CastU16En4/1
  CastU16En3/1 -> Switch/3, Saturation/1
  CastU16En4/1 -> CastU16En3/1
  LTEp25/1 -> QuadHandle2/2
  LTEp50/1 -> QuadHandle1/2, RAMDelayBalance/1
  PipelineRegister/1 -> Positive/1, Negate/1
  Negate/1 -> SignCorrected/3
  Point25/1 -> LTEp25/2
  Point50/1 -> p50mA/1, LTEp50/2, Amp50/2
  Positive/1 -> SignCorrected/1
  QuadHandle1/1 -> p50mA/2, QuadHandle2/1, LTEp25/1
  QuadHandle2/1 -> CastU16En2/1
  delayMatch/1 -> SignCorrected/2
  Saturation/1 -> Switch/1
  SignCorrected/1 -> Sine/1
  Switch/1 -> Look-Up Table/1
  insig/1 -> QuadHandle1/1, LTEp50/1, Amp50/1
  p50mA/1 -> QuadHandle2/3
  pow2switch/1 -> Switch/2
  u/1 -> insig/1
  RAMDelayBalance/1 -> delayMatch/1
  Look-Up Table/1 -> PipelineRegister/1

== system gm_Tx_OFDM/Transmitter/OFDM Modulator/OFDM Modulator ==
  data : Inport  OutDataTypeStr=fixdt(1,16,14,'DataTypeOverride', 'Off')  PortDimensions=[64]  SampleTime=0.0064
      settings: SignalType=complex
  valid : Inport  Port=2  OutDataTypeStr=boolean  SampleTime=0.0064
  OFDM Modulator : whdlmod/OFDM Modulator  OFDMParametersSource=Property  FFTLength=N*2  MaxFFTLength=64  CPLength=32  numLgSc=16  numRgSc=15  InsertDCNull=on  Windowing=off  WindowLength=8  MaxWindowLength=8  ResetInputPort=off  Normalize=on  RoundingMethod=Floor  SimulateUsing=Code generation
  OFDM Modulator_term1 : Terminator
  OFDM Modulator_term2 : Terminator
  data1 : Outport  SampleTime=0.0064
  wires:
  OFDM Modulator/1 -> data1/1
  OFDM Modulator/2 -> OFDM Modulator_term1/1
  OFDM Modulator/3 -> OFDM Modulator_term2/1
  data/1 -> OFDM Modulator/1
  valid/1 -> OFDM Modulator/2

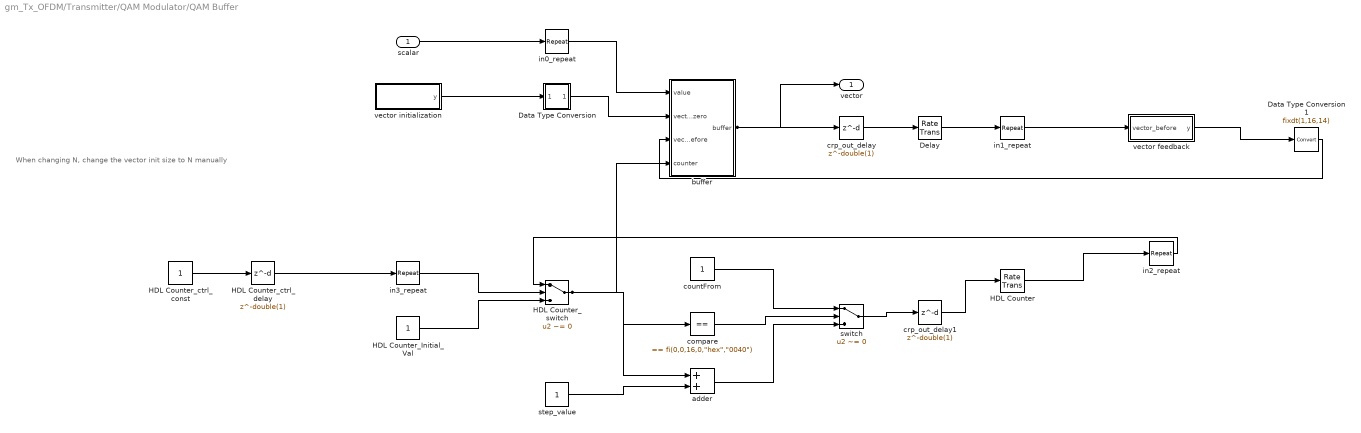
== system gm_Tx_OFDM/Transmitter/QAM Modulator/QAM Buffer ==
  note: When changing N, change the vector init size to N manually
  scalar : Inport  OutDataTypeStr=fixdt(1, 16, 13)  PortDimensions=1  SampleTime=0.0001
      settings: SignalType=complex
  Data Type Conversion : Subsystem
      mask Display: disp('NFP\nconv');
  Data Type Conversion1 : DataTypeConversion  OutDataTypeStr=fixdt(1,16,14)
  Delay : RateTransition  OutPortSampleTimeOpt=Multiple of input port sample time  OutPortSampleTimeMultiple=64
  HDL Counter : RateTransition  OutPortSampleTimeOpt=Multiple of input port sample time  OutPortSampleTimeMultiple=64
  HDL Counter_Initial_Val : Constant  OutDataTypeStr=uint16  SampleTime=1.5625e-06
  HDL Counter_ctrl_const : Constant  OutDataTypeStr=boolean  SampleTime=0.0001
  HDL Counter_ctrl_delay : Delay  DelayLength=double(1)  InitialCondition=0  SampleTime=0.0001
  HDL Counter_switch : Switch  Criteria=u2 ~= 0  Threshold=double(0)  OutDataTypeStr=uint16  SampleTime=1.5625e-06  SaturateOnIntegerOverflow=off  InputSameDT=off
  adder : Sum  AccumDataTypeStr=uint16  OutDataTypeStr=uint16  SampleTime=1.5625e-06
  buffer : Subsystem
  compare : simulink/Logic and Bit Operations/Compare To Constant  relop===  const="fi(0,0,16,0,\"hex\",\"0040\")"  OutDataTypeStr=boolean
  countFrom : Constant  VectorParams1D=off  OutDataTypeStr=uint16  SampleTime=1.5625e-06
  crp_out_delay : Delay  DelayLength=double(1)  InitialCondition=0  SampleTime=1.5625e-06
  crp_out_delay1 : Delay  DelayLength=double(1)  InitialCondition=0  SampleTime=1.5625e-06
  in0_repeat : dspsigops/Repeat  FactorSource=Dialog parameter  N=double(64)  Nmax=16  RateOptions=Allow multirate processing  ic=0  mode=Unused parameter value
  in1_repeat : dspsigops/Repeat  FactorSource=Dialog parameter  N=double(64)  Nmax=16  RateOptions=Allow multirate processing  ic=0  mode=Unused parameter value
  in2_repeat : dspsigops/Repeat  FactorSource=Dialog parameter  N=double(64)  Nmax=16  RateOptions=Allow multirate processing  ic=0  mode=Unused parameter value
  in3_repeat : dspsigops/Repeat  FactorSource=Dialog parameter  N=double(64)  Nmax=16  RateOptions=Allow multirate processing  ic=0  mode=Unused parameter value
  step_value : Constant  VectorParams1D=off  OutDataTypeStr=uint16  SampleTime=1.5625e-06
  switch : Switch  Criteria=u2 ~= 0  Threshold=double(0)  OutDataTypeStr=uint16  SampleTime=1.5625e-06  SaturateOnIntegerOverflow=off  InputSameDT=off
  vector feedback : Subsystem
  vector initialization : Subsystem
  vector : Outport  SampleTime=1.5625e-06
  wires:
  HDL Counter_ctrl_delay/1 -> in3_repeat/1
  HDL Counter_ctrl_const/1 -> HDL Counter_ctrl_delay/1
  buffer/1(buffer) -> vector/1, crp_out_delay/1
  in0_repeat/1 -> buffer/1(value)
  in3_repeat/1 -> HDL Counter_switch/2
  scalar/1 -> in0_repeat/1
  HDL Counter/1 -> in2_repeat/1
  in2_repeat/1 -> HDL Counter_switch/1
  Delay/1 -> in1_repeat/1
  in1_repeat/1 -> vector feedback/1(vector_before)
  crp_out_delay/1 -> Delay/1
  crp_out_delay1/1 -> HDL Counter/1
  vector feedback/1(y) -> Data Type Conversion1/1
  Data Type Conversion1/1 -> buffer/3(vector_before)
  countFrom/1 -> switch/1
  step_value/1 -> adder/2
  adder/1 -> switch/3
  switch/1 -> crp_out_delay1/1
  compare/1 -> switch/2
  HDL Counter_Initial_Val/1 -> HDL Counter_switch/3
  HDL Counter_switch/1 -> compare/1, adder/1, buffer/4(counter)
  vector initialization/1(y) -> Data Type Conversion/1(In1)
  Data Type Conversion/1(Out1) -> buffer/2(vector_zero)

== system gm_Tx_OFDM/Transmitter/IQ Modulator/Cosine Debuffer/debuffer ==
  vector_in : Inport  OutDataTypeStr=fixdt(1, 16, 14)  PortDimensions=[64 1]  SampleTime=1.5625e-06
  counter : Inport  Port=2  OutDataTypeStr=int16  PortDimensions=1  SampleTime=1.5625e-06
  vector_before : Inport  Port=3  OutDataTypeStr=fixdt(1, 16, 14)  PortDimensions=[64]  SampleTime=1.5625e-06
  debuffer : MATLAB Function  TreatAsAtomicUnit=on
  zp : Subsystem
  buffer : Outport  SampleTime=1.5625e-06
  vector_current : Outport  Port=2  SampleTime=1.5625e-06
  wires:
  debuffer/1(buffer) -> buffer/1
  debuffer/2(vector_current) -> vector_current/1
  vector_in/1 -> debuffer/1(vector_in)
  counter/1 -> zp/1(in0)
  vector_before/1 -> debuffer/3(vector_before)
  zp/1(out0) -> debuffer/2(counter)

== system gm_Tx_OFDM/Transmitter/IQ Modulator/Cosine Debuffer1/debuffer ==
  vector_in : Inport  OutDataTypeStr=fixdt(1, 16, 14)  PortDimensions=[64 1]  SampleTime=1.5625e-06
  counter : Inport  Port=2  OutDataTypeStr=int16  PortDimensions=1  SampleTime=1.5625e-06
  vector_before : Inport  Port=3  OutDataTypeStr=fixdt(1, 16, 14)  PortDimensions=[64]  SampleTime=1.5625e-06
  debuffer : MATLAB Function  TreatAsAtomicUnit=on
  zp : Subsystem
  buffer : Outport  SampleTime=1.5625e-06
  vector_current : Outport  Port=2  SampleTime=1.5625e-06
  wires:
  debuffer/1(buffer) -> buffer/1
  debuffer/2(vector_current) -> vector_current/1
  vector_in/1 -> debuffer/1(vector_in)
  counter/1 -> zp/1(in0)
  vector_before/1 -> debuffer/3(vector_before)
  zp/1(out0) -> debuffer/2(counter)

== system gm_Tx_OFDM/Transmitter/QAM Modulator/QAM Buffer/Data Type Conversion ==
  In1 : Inport
  Data Type Conversion : DataTypeConversion  OutDataTypeStr=fixdt(1, 16, 14)  SampleTime=1.5625e-06  SaturateOnIntegerOverflow=off  RndMeth=Floor
  Data Type Conversion_pd1 : Delay  DelayLength=6
  Out1 : Outport
  wires:
  In1/1 -> Data Type Conversion/1
  Data Type Conversion/1 -> Data Type Conversion_pd1/1
  Data Type Conversion_pd1/1 -> Out1/1

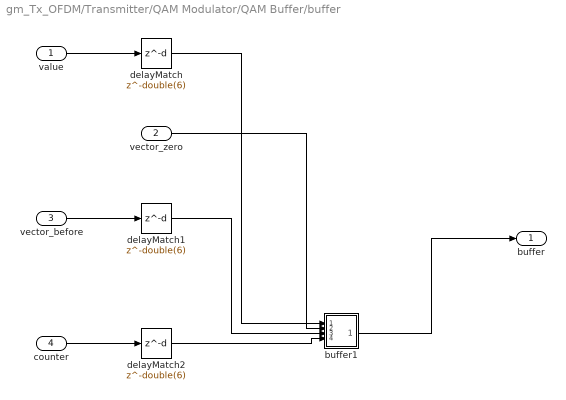
== system gm_Tx_OFDM/Transmitter/QAM Modulator/QAM Buffer/buffer ==
  value : Inport  OutDataTypeStr=fixdt(1, 16, 13)  PortDimensions=1  SampleTime=1.5625e-06
      settings: SignalType=complex
  vector_zero : Inport  Port=2  OutDataTypeStr=fixdt(1, 16, 14)  PortDimensions=[64]  SampleTime=1.5625e-06
      settings: SignalType=complex
  vector_before : Inport  Port=3  OutDataTypeStr=fixdt(1, 16, 14)  PortDimensions=[64]  SampleTime=1.5625e-06
      settings: SignalType=complex
  counter : Inport  Port=4  OutDataTypeStr=uint16  PortDimensions=1  SampleTime=1.5625e-06
  buffer1 : MATLAB Function  TreatAsAtomicUnit=on
  delayMatch : Delay  DelayLength=double(6)  InitialCondition=0  SampleTime=1.5625e-06
  delayMatch1 : Delay  DelayLength=double(6)  InitialCondition=0  SampleTime=1.5625e-06
  delayMatch2 : Delay  DelayLength=double(6)  InitialCondition=0  SampleTime=1.5625e-06
  buffer : Outport  SampleTime=1.5625e-06
  wires:
  buffer1/1(buffer) -> buffer/1
  delayMatch/1 -> buffer1/1(value)
  delayMatch1/1 -> buffer1/3(vector_before)
  delayMatch2/1 -> buffer1/4(counter)
  value/1 -> delayMatch/1
  vector_zero/1 -> buffer1/2(vector_zero)
  vector_before/1 -> delayMatch1/1
  counter/1 -> delayMatch2/1

== system gm_Tx_OFDM/Transmitter/QAM Modulator/QAM Buffer/vector feedback ==
  vector_before : Inport  OutDataTypeStr=fixdt(1, 16, 14)  PortDimensions=[64]  SampleTime=1.5625e-06
      settings: SignalType=complex
  vector feedback : MATLAB Function  TreatAsAtomicUnit=on
  y : Outport  SampleTime=1.5625e-06  VectorParamsAs1DForOutWhenUnconnected=off
  wires:
  vector feedback/1(y) -> y/1
  vector_before/1 -> vector feedback/1(vector_before)

== system gm_Tx_OFDM/Transmitter/QAM Modulator/QAM Buffer/vector initialization ==
  Reshape : Reshape
  const : Constant  Value="repmat(complex(1, 0),[64   1])"  VectorParams1D=off  OutDataTypeStr=double  SampleTime=1.5625e-06
  y : Outport  SampleTime=1.5625e-06  VectorParamsAs1DForOutWhenUnconnected=off
  wires:
  Reshape/1 -> y/1
  const/1 -> Reshape/1

== system gm_Tx_OFDM/Transmitter/IQ Modulator/Cosine Debuffer/debuffer/zp ==
  in0 : Inport  OutDataTypeStr=fixdt(1,16,0,'DataTypeOverride', 'Off')  SampleTime=1.5625e-06
  t : Constant  Value=double(1)  OutDataTypeStr=int16  SampleTime=1.5625e-06
  t1 : Switch  Threshold=double(1)  OutDataTypeStr=int16  SampleTime=1.5625e-06  SaturateOnIntegerOverflow=off  InputSameDT=off
  out0 : Outport  OutDataTypeStr=int16  SampleTime=1.5625e-06
  wires:
  t/1 -> t1/3
  t1/1 -> out0/1
  in0/1 -> t1/1, t1/2

== system gm_Tx_OFDM/Transmitter/IQ Modulator/Cosine Debuffer1/debuffer/zp ==
  in0 : Inport  OutDataTypeStr=fixdt(1,16,0,'DataTypeOverride', 'Off')  SampleTime=1.5625e-06
  t : Constant  Value=double(1)  OutDataTypeStr=int16  SampleTime=1.5625e-06
  t1 : Switch  Threshold=double(1)  OutDataTypeStr=int16  SampleTime=1.5625e-06  SaturateOnIntegerOverflow=off  InputSameDT=off
  out0 : Outport  OutDataTypeStr=int16  SampleTime=1.5625e-06
  wires:
  t/1 -> t1/3
  t1/1 -> out0/1
  in0/1 -> t1/1, t1/2

== matlab function gm_Tx_OFDM/Receiver/FFT Debuffer/vector feedback ==
  data: y output; vector_before input
function y = fcn(vector_before)
%#codegen

y = complex(vector_before);

== matlab function gm_Tx_OFDM/Transmitter/IQ Modulator/Cosine Debuffer1/debuffer/debuffer ==
  data: vector_in input; buffer output; counter input; vector_current output; vector_before input size=64
function [buffer, vector_current]= fcn(vector_in, counter, vector_before)
%#codegen

if(counter == 1)
    vector_current = vector_in;
else
    vector_current = vector_before;
end

buffer = vector_current(counter);

== matlab function gm_Tx_OFDM/Receiver/Rx Buffer/buffer ==
  data: value input; vector_zero input; vector_before input; counter input; buffer output
function buffer = fcn(value, vector_zero, vector_before, counter)
%#codegen
if(counter == 0)
    buffer = vector_zero;
else
    buffer = vector_before;
end

buffer(counter) = value;

== matlab function gm_Tx_OFDM/Transmitter/QAM Modulator/QAM Buffer/buffer/buffer1 ==
  data: value input; vector_zero input; vector_before input; counter input; buffer output
function buffer = fcn(value, vector_zero, vector_before, counter)
%#codegen
if(counter == 0)
    buffer = vector_zero;
else
    buffer = vector_before;
end

buffer(counter) = value;

== matlab function gm_Tx_OFDM/Transmitter/QAM Modulator/QAM Buffer/vector feedback/vector feedback ==
  data: y output; vector_before input
function y = fcn(vector_before)
%#codegen

y = complex(vector_before);

== matlab function gm_Tx_OFDM/Receiver/Rx Buffer/vector feedback ==
  data: y output; vector_before input
function y = fcn(vector_before)
%#codegen

y = (vector_before);

== matlab function gm_Tx_OFDM/Transmitter/IQ Modulator/Cosine Debuffer/debuffer/debuffer ==
  data: vector_in input; buffer output; counter input; vector_current output; vector_before input size=64
function [buffer, vector_current]= fcn(vector_in, counter, vector_before)
%#codegen

if(counter == 1)
    vector_current = vector_in;
else
    vector_current = vector_before;
end

buffer = vector_current(counter);

== matlab function gm_Tx_OFDM/Receiver/Rx Buffer/vector initialization ==
  data: y output
function y = fcn()
%#codegen

y = (ones(64,1));

== matlab function gm_Tx_OFDM/Receiver/IQ Demodulator/Hilbert Transform ==
  data: u input; y output
function y = fcn(u)
%#codegen

u = cast(u, "double");
Q = hilbert(u);

y = imag(u);

== matlab function gm_Tx_OFDM/Receiver/IQ Demodulator/Sine memory ==
  data: y output
function y = fcn()
%#codegen

y = [
0.0
0.098017
0.19509
0.290285
0.382683
0.471397
0.55557
0.634393
0.707107
0.77301
0.83147
0.881921
0.92388
0.95694
0.980785
0.995185
1
0.995185
0.980785
0.95694
0.92388
0.881921
0.83147
0.77301
0.707107
0.634393
0.55557
0.471397
0.382683
0.290285
0.19509
0.098017
0.0
-0.098017
-0.19509
-0.290285
-0.382683
-0.471397
-0.55557
-0.634393
-0.707107
-0.77301
-0.83147
-0.881921
-0.92388
-0.95694
-0.980785
-0.995185
-1.0
-0.995185
-0.980785
-0.95694
-0.92388
-0.881921
-0.83147
-0.77301
-0.707107
-0.634393
-0.55557
-0.471397
-0.382683
-0.290285
-0.19509
-0.098017    
];

== matlab function gm_Tx_OFDM/Receiver/IQ Demodulator/Cosine memory ==
  data: y output
function y = fcn()
%#codegen

y = [
1
0.995185
0.980785
0.95694
0.92388
0.881921
0.83147
0.77301
0.707107
0.634393
0.55557
0.471397
0.382683
0.290285
0.19509
0.098017
0.0
-0.098017
-0.19509
-0.290285
-0.382683
-0.471397
-0.55557
-0.634393
-0.707107
-0.77301
-0.83147
-0.881921
-0.92388
-0.95694
-0.980785
-0.995185
-1.0
-0.995185
-0.980785
-0.95694
-0.92388
-0.881921
-0.83147
-0.77301
-0.707107
-0.634393
-0.55557
-0.471397
-0.382683
-0.290285
-0.19509
-0.098017
-0.0
0.098017
0.19509
0.290285
0.382683
0.471397
0.55557
0.634393
0.707107
0.77301
0.83147
0.881921
0.92388
0.95694
0.980785
0.995185    
];

== matlab function gm_Tx_OFDM/Receiver/IQ Demodulator/Minus Sine memory ==
  data: y output
function y = fcn()
%#codegen

y = [
0.0
0.098017
0.19509
0.290285
0.382683
0.471397
0.55557
0.634393
0.707107
0.77301
0.83147
0.881921
0.92388
0.95694
0.980785
0.995185
1
0.995185
0.980785
0.95694
0.92388
0.881921
0.83147
0.77301
0.707107
0.634393
0.55557
0.471397
0.382683
0.290285
0.19509
0.098017
0.0
-0.098017
-0.19509
-0.290285
-0.382683
-0.471397
-0.55557
-0.634393
-0.707107
-0.77301
-0.83147
-0.881921
-0.92388
-0.95694
-0.980785
-0.995185
-1.0
-0.995185
-0.980785
-0.95694
-0.92388
-0.881921
-0.83147
-0.77301
-0.707107
-0.634393
-0.55557
-0.471397
-0.382683
-0.290285
-0.19509
-0.098017    
];

== matlab function gm_Tx_OFDM/Receiver/FFT Debuffer/debuffer ==
  data: vector_in input; buffer output; counter input; vector_current output; vector_before input size=64
function [buffer, vector_current]= fcn(vector_in, counter, vector_before)
%#codegen

if(counter == 1)
    vector_current = vector_in;
else
    vector_current = vector_before;
end

buffer = vector_current(counter);
